simulink model "motor"  (R2024a)
settings: Solver=VariableStepAuto  StartTime=0.0  StopTime=0.1  RelTol=1e-3
PreLoadFcn:
  | run("values.m")
values from neighbouring files (symbols this model uses):
  I = 3.39*10^(-3)    (= 0.00339)    [values.m]
  J = 3.88*10^(-5)    (= 3.88e-05)    [values.m]
  Kt = 0.056    [values.m]
  Rl = 0.8    [values.m]
  Rr = 0.35    [values.m]
  Rt = 1.1e-4    (= 0.00011)    [values.m]
settings Model: Creator=hansf  LastModifiedBy=danfr755
settings RTWCC: GPUComputeCapability=3.5

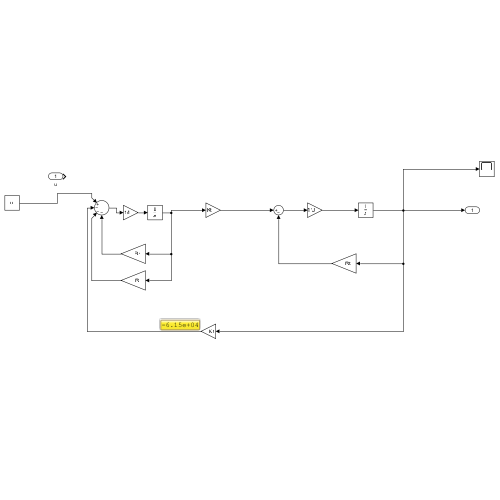
[thumbnail: Simulink's stored preview of the top-level diagram]
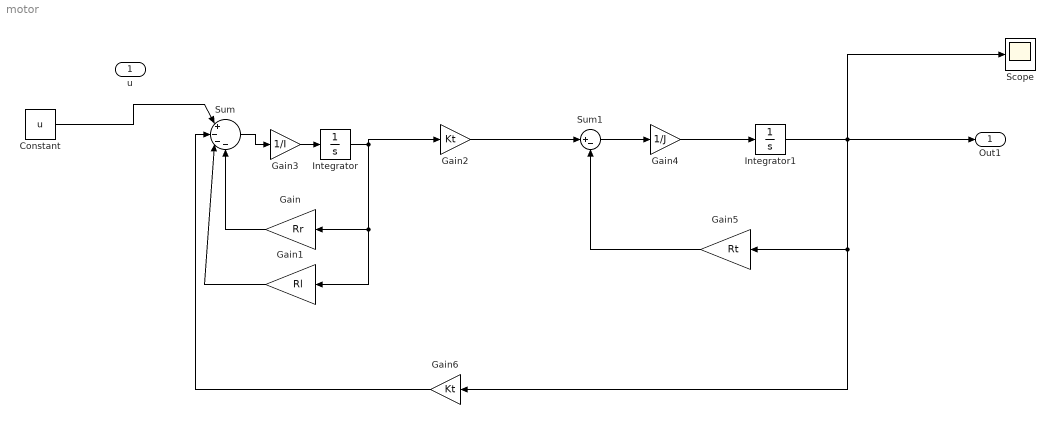
== system motor ==
  u : Inport
  Constant : Constant  Value=u
  Gain : Gain  Gain=Rr
  Gain1 : Gain  Gain=Rl
  Gain2 : Gain  Gain=Kt
  Gain3 : Gain  Gain=1/I
  Gain4 : Gain  Gain=1/J
  Gain5 : Gain  Gain=Rt
  Gain6 : Gain  Gain=Kt
  Integrator : Integrator
  Integrator1 : Integrator
  Scope : Scope
  Sum : Sum  Inputs=|+---
  Sum1 : Sum  Inputs=|+-
  Out1 : Outport
  wires:
  Integrator/1 -> Gain2/1, Gain1/1, Gain/1
  Gain2/1 -> Sum1/1
  Sum/1 -> Gain3/1
  Gain3/1 -> Integrator/1
  Sum1/1 -> Gain4/1
  Gain4/1 -> Integrator1/1
  Constant/1 -> Sum/1
  Integrator1/1 -> Gain6/1, Gain5/1, Scope/1, Out1/1
  Gain6/1 -> Sum/2
  Gain/1 -> Sum/4
  Gain1/1 -> Sum/3
  Gain5/1 -> Sum1/2
